simulink model "ACCMod003_dist"  (Simulink 8.3)
settings: Solver=FixedStepDiscrete  StartTime=0.0  StopTime=10.0  FixedStep=0.1  RelTol=1e-3
model workspace (MAT data in the model file):
  pACC.Kp = 0.5
  pACC.minDist2Target = 50
  pACC.avgACCactiveTime = 20
  pACC.LearnGain = 10
  pACC.Ki = 1e-05
  pACC.KpDist = 1
  pACC.KiDist = 0.01
  pACC.SampleTime = 0.1
  pACC.ACCBuffer : numeric (value not decoded)
libraries: Lib_Controls x4, simulink x1
settings Model: Creator=swami  LastModifiedBy=swami
settings DataIOCC: SignalLoggingSaveFormat=Dataset
settings DebuggingCC: UnderspecifiedInitializationDetection=Simplified  StateNameClashWarn=none
settings GRTTargetCC: CombineOutputUpdateFcns=on  GRTInterface=off

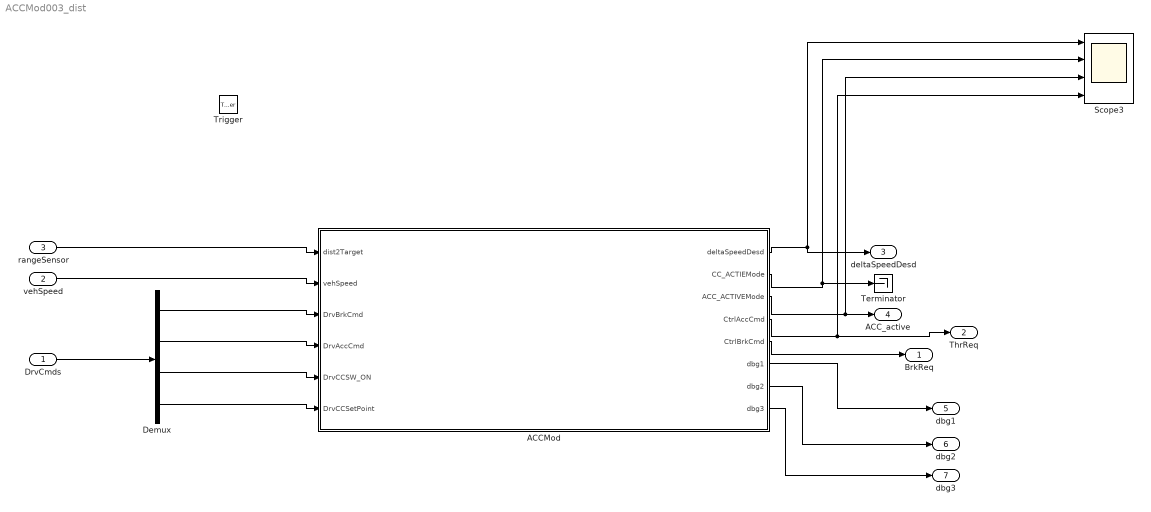
== system ACCMod003_dist ==
  DrvCmds : Inport  PortDimensions=4
  vehSpeed : Inport  Port=2
  rangeSensor : Inport  Port=3
  Trigger : TriggerPort  TriggerType=function-call  PortDimensions=1
  ACCMod : Subsystem  mask{minDist2TargetCal=pACC.minDist2Target, ACCBuffer=pACC.ACCBuffer, Kp=pACC.Kp, Ki=pACC.Ki, KpDist=pACC.KpDist, KiDist=pACC.KiDist, SampleTime=pACC.SampleTime, LearnGain=pACC.LearnGain, avgACCactiveTime=pACC.avgACCactiveTime}
      mask prompts: minDist2TargetCal "minDist2Target"
  Demux : Demux
  Scope3 : Scope  NumInputPorts=4
      settings: TimeRange=50  YMin=-5~-5~-5~-5  YMax=5~5~5~5  SaveName=ScopeData4
  Terminator : Terminator
  BrkReq : Outport  PortDimensions=1
  ThrReq : Outport  Port=2  PortDimensions=1
  deltaSpeedDesd : Outport  Port=3  PortDimensions=1
  ACC_active : Outport  Port=4  PortDimensions=1
  dbg1 : Outport  Port=5  PortDimensions=1
  dbg2 : Outport  Port=6  PortDimensions=1
  dbg3 : Outport  Port=7  PortDimensions=1
  wires:
  DrvCmds/1 -> Demux/1
  Demux/3 -> ACCMod/5(DrvCCSW_ON)
  Demux/4 -> ACCMod/6(DrvCCSetPoint)
  rangeSensor/1 -> ACCMod/1(dist2Target)
  vehSpeed/1 -> ACCMod/2(vehSpeed)
  ACCMod/3(ACC_ACTIVEMode) -> Scope3/3, ACC_active/1
  ACCMod/5(CtrlBrkCmd) -> BrkReq/1
  ACCMod/1(deltaSpeedDesd) -> Scope3/1, deltaSpeedDesd/1
  ACCMod/4(CtrlAccCmd) -> ThrReq/1, Scope3/4
  ACCMod/2(CC_ACTIEMode) -> Scope3/2, Terminator/1
  Demux/1 -> ACCMod/3(DrvBrkCmd)
  Demux/2 -> ACCMod/4(DrvAccCmd)
  ACCMod/6(dbg1) -> dbg1/1
  ACCMod/7(dbg2) -> dbg2/1
  ACCMod/8(dbg3) -> dbg3/1

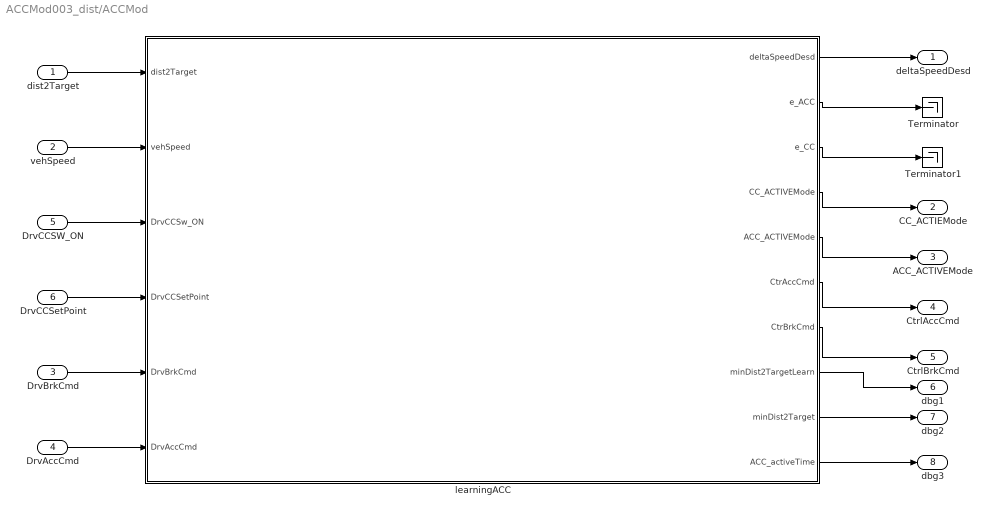
== system ACCMod003_dist/ACCMod ==
  dist2Target : Inport
  vehSpeed : Inport  Port=2
  DrvBrkCmd : Inport  Port=3
  DrvAccCmd : Inport  Port=4
  DrvCCSW_ON : Inport  Port=5
  DrvCCSetPoint : Inport  Port=6
  Terminator : Terminator
  Terminator1 : Terminator
  learningACC : Stateflow chart  TreatAsAtomicUnit=on
  deltaSpeedDesd : Outport
  CC_ACTIEMode : Outport  Port=2
  ACC_ACTIVEMode : Outport  Port=3
  CtrlAccCmd : Outport  Port=4
  CtrlBrkCmd : Outport  Port=5
  dbg1 : Outport  Port=6
  dbg2 : Outport  Port=7
  dbg3 : Outport  Port=8
  wires:
  DrvCCSetPoint/1 -> learningACC/4(DrvCCSetPoint)
  DrvAccCmd/1 -> learningACC/6(DrvAccCmd)
  DrvCCSW_ON/1 -> learningACC/3(DrvCCSw_ON)
  dist2Target/1 -> learningACC/1(dist2Target)
  learningACC/5(" ACC_ACTIVEMode") -> ACC_ACTIVEMode/1
  learningACC/1(deltaSpeedDesd) -> deltaSpeedDesd/1
  learningACC/4(" CC_ACTIVEMode") -> CC_ACTIEMode/1
  DrvBrkCmd/1 -> learningACC/5(DrvBrkCmd)
  vehSpeed/1 -> learningACC/2(vehSpeed)
  learningACC/6(CtrAccCmd) -> CtrlAccCmd/1
  learningACC/7(CtrBrkCmd) -> CtrlBrkCmd/1
  learningACC/2(e_ACC) -> Terminator/1
  learningACC/3(e_CC) -> Terminator1/1
  learningACC/8(minDist2TargetLearn) -> dbg1/1
  learningACC/9(minDist2Target) -> dbg2/1
  learningACC/10(ACC_activeTime) -> dbg3/1

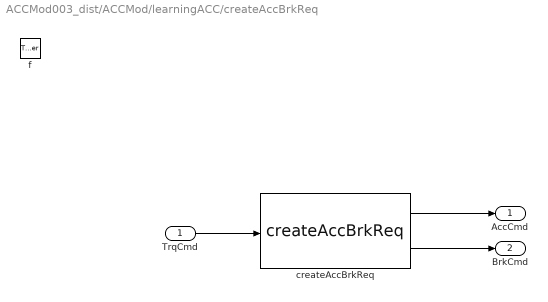
== system ACCMod003_dist/ACCMod/learningACC/createAccBrkReq ==
  TrqCmd : Inport  OutDataTypeStr=double  PortDimensions=1
  f : TriggerPort  TriggerType=function-call
      settings: CopyFcn=Stateflow.SLINSF.SimulinkMan.removeBlockPreDeleteFcn  PreDeleteFcn=Stateflow.SLINSF.SimulinkMan.unsafePredeleteFcn
  createAccBrkReq : Lib_Controls/createAccBrkReq
  AccCmd : Outport
  BrkCmd : Outport  Port=2
  wires:
  TrqCmd/1 -> createAccBrkReq/1
  createAccBrkReq/1 -> AccCmd/1
  createAccBrkReq/2 -> BrkCmd/1

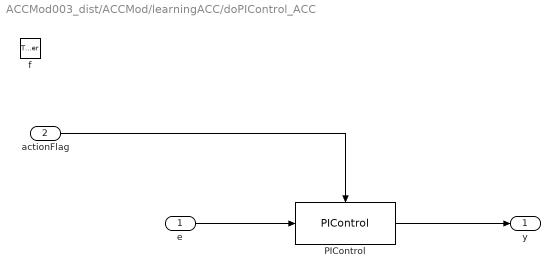
== system ACCMod003_dist/ACCMod/learningACC/doPIControl_ACC ==
  e : Inport  OutDataTypeStr=double  PortDimensions=1
  actionFlag : Inport  Port=2  OutDataTypeStr=double  PortDimensions=1
  f : TriggerPort  TriggerType=function-call
      settings: CopyFcn=Stateflow.SLINSF.SimulinkMan.removeBlockPreDeleteFcn  PreDeleteFcn=Stateflow.SLINSF.SimulinkMan.unsafePredeleteFcn
  PIControl : Lib_Controls/PIControl  Kp=KpDist  Ki=KiDist
  y : Outport
  wires:
  PIControl/1 -> y/1
  e/1 -> PIControl/1
  actionFlag/1 -> PIControl/Enable

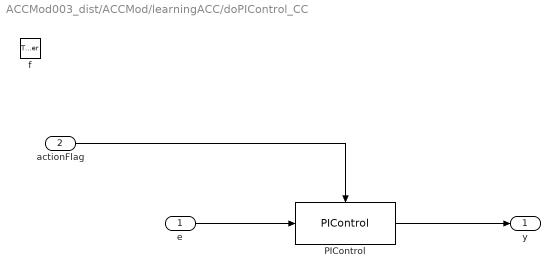
== system ACCMod003_dist/ACCMod/learningACC/doPIControl_CC ==
  e : Inport  OutDataTypeStr=double  PortDimensions=1
  actionFlag : Inport  Port=2  OutDataTypeStr=double  PortDimensions=1
  f : TriggerPort  TriggerType=function-call
      settings: CopyFcn=Stateflow.SLINSF.SimulinkMan.removeBlockPreDeleteFcn  PreDeleteFcn=Stateflow.SLINSF.SimulinkMan.unsafePredeleteFcn
  PIControl : Lib_Controls/PIControl  Kp=Kp  Ki=Ki
      link override Constant: Value=0
  y : Outport
  wires:
  PIControl/1 -> y/1
  e/1 -> PIControl/1
  actionFlag/1 -> PIControl/Enable

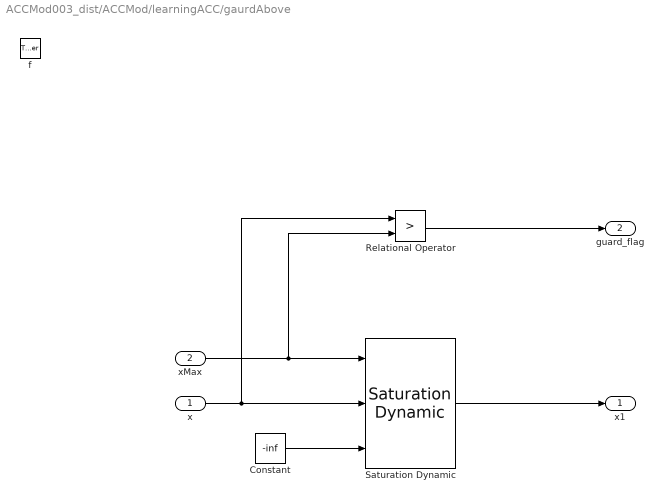
== system ACCMod003_dist/ACCMod/learningACC/gaurdAbove ==
  x : Inport  OutDataTypeStr=double  PortDimensions=1
  xMax : Inport  Port=2  OutDataTypeStr=double  PortDimensions=1
  f : TriggerPort  TriggerType=function-call
      settings: CopyFcn=Stateflow.SLINSF.SimulinkMan.removeBlockPreDeleteFcn  PreDeleteFcn=Stateflow.SLINSF.SimulinkMan.unsafePredeleteFcn
  Constant : Constant  Value=-inf
  Relational Operator : RelationalOperator  Operator=>  OutDataTypeStr=boolean
  Saturation Dynamic : simulink/Discontinuities/Saturation Dynamic  OutMin=[]  OutMax=[]  OutDataTypeStr=Inherit: Same as second input  OutDataType=fixdt(1, 16)  OutScaling=2^-10  DoSatur=off
  x1 : Outport
  guard_flag : Outport  Port=2
  wires:
  xMax/1 -> Relational Operator/2, Saturation Dynamic/1
  x/1 -> Relational Operator/1, Saturation Dynamic/2
  Constant/1 -> Saturation Dynamic/3
  Saturation Dynamic/1 -> x1/1
  Relational Operator/1 -> guard_flag/1

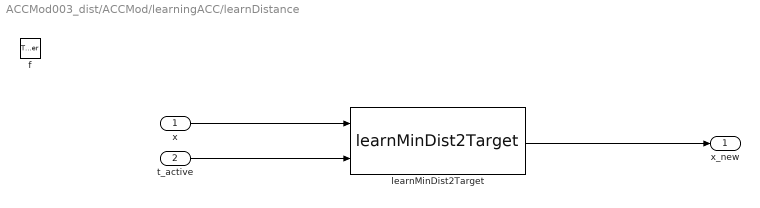
== system ACCMod003_dist/ACCMod/learningACC/learnDistance ==
  x : Inport  OutDataTypeStr=double  PortDimensions=1
  t_active : Inport  Port=2  OutDataTypeStr=double  PortDimensions=1
  f : TriggerPort  TriggerType=function-call
      settings: CopyFcn=Stateflow.SLINSF.SimulinkMan.removeBlockPreDeleteFcn  PreDeleteFcn=Stateflow.SLINSF.SimulinkMan.unsafePredeleteFcn
  learnMinDist2Target : Lib_Controls/learnMinDist2Target
  x_new : Outport
  wires:
  x/1 -> learnMinDist2Target/1
  t_active/1 -> learnMinDist2Target/2
  learnMinDist2Target/1 -> x_new/1

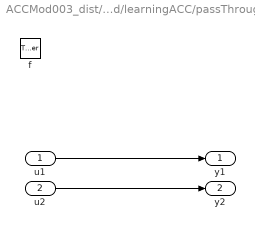
== system ACCMod003_dist/ACCMod/learningACC/passThrough ==
  u1 : Inport  OutDataTypeStr=double  PortDimensions=1
  u2 : Inport  Port=2  OutDataTypeStr=double  PortDimensions=1
  f : TriggerPort  TriggerType=function-call
      settings: CopyFcn=Stateflow.SLINSF.SimulinkMan.removeBlockPreDeleteFcn  PreDeleteFcn=Stateflow.SLINSF.SimulinkMan.unsafePredeleteFcn
  y1 : Outport
  y2 : Outport  Port=2
  wires:
  u1/1 -> y1/1
  u2/1 -> y2/1

== stateflow chart ACCMod/learningACC ==
  state CC_ACTIVE
    entry:
    deltaSpeedDesd = 0;
    e_CC = (DrvCCSetPoint + deltaSpeedDesd - vehSpeed);
    doPIControl_CC(e_CC,startAction);
    minDist2TargetLearn = 0;
    during:
    e_CC = (DrvCCSetPoint + deltaSpeedDesd - vehSpeed);
    [CtrAccCmd, CtrBrkCmd]  = createAccBrkReq(doPIControl_CC(e_CC,doAction));
    exit:
    [CtrAccCmd, CtrBrkCmd]  = createAccBrkReq(doPIControl_CC(e_CC,stopAction));
    state ACC_ACTIVE
      entry:
      e_ACC = dist2Target - minDist2Target;
      doPIControl_ACC(e_ACC,startAction);
      ACC_activeTime = 0;
      during:
      minDist2Target = minDist2TargetCal + minDist2TargetLearn;
      ACC_activeTime = ACC_activeTime + SampleTime;
      e_ACC = dist2Target - minDist2Target;
      deltaSpeedDesd = doPIControl_ACC(e_ACC,doAction);
      [deltaSpeedDesd, turn_ACC_OFF] = gaurdAbove(deltaSpeedDesd, 0);
      exit:
      minDist2TargetLearn = learnDistance(minDist2TargetLearn, ...
      ACC_activeTime);
    state ACC_INACTIVE
      entry:
      deltaSpeedDesd = 0;
      during:
      minDist2Target = minDist2TargetCal + minDist2TargetLearn;
    (default) -> ACC_INACTIVE
    ACC_ACTIVE -> ACC_INACTIVE [order 2] : [turn_ACC_OFF]
    ACC_ACTIVE -> ACC_INACTIVE [order 1] : [dist2Target>(minDist2Target)]
    ACC_INACTIVE -> ACC_ACTIVE : [dist2Target < minDist2Target]
  state CC_INACTIVE
    entry:
    minDist2TargetLearn = 0;
    during:
    [CtrAccCmd, CtrBrkCmd] = passThrough(DrvAccCmd, DrvBrkCmd);
  state [y1,y2] = passThrough(u1,u2) [function]
  state y = doPIControl_CC(e,actionFlag) [function]
  state [AccCmd, BrkCmd] = createAccBrkReq(TrqCmd) [function]
  state y = doPIControl_ACC(e,actionFlag) [function]
  state x_new = learnDistance(x,t_active) [function]
  state [x1, guard_flag] = gaurdAbove(x,xMax) [function]
  (default) -> CC_INACTIVE
  CC_ACTIVE -> CC_INACTIVE : [DrvCCSw_ON<0.5]
  CC_INACTIVE -> CC_ACTIVE : [DrvCCSw_ON>0.5]
  data: u1 function_input double size=1; u2 function_input double size=1; y1 function_output double; y2 function_output double; e function_input double size=1; y function_output double; actionFlag function_input double size=1; TrqCmd function_input double size=1; AccCmd function_output double; BrkCmd function_output double; e function_input double size=1; y function_output double; actionFlag function_input double size=1; x_new function_output double; x function_input double size=1; t_active function_input double size=1; x function_input double size=1; x1 function_output double; guard_flag function_output double; xMax function_input double size=1; minDist2TargetCal parameter double; dist2Target input double; ACCBuffer parameter double; turn_ACC_OFF local double; vehSpeed input double; DrvCCSw_ON input double; deltaSpeedDesd output double; e_ACC output double; e_CC output double; CC_ACTIVEMode output boolean; ACC_ACTIVEMode output boolean; DrvCCSetPoint input double; DrvBrkCmd input double; DrvAccCmd input double; CtrAccCmd output double; CtrBrkCmd output double; stopAction constant double =0; doAction constant double =2; startAction constant double =1; minDist2TargetLearn output double; minDist2Target output double; SampleTime parameter double; ACC_activeTime output double
